simulink model "flightSimulator2"  (R2022a)
settings: Solver=VariableStepAuto  StartTime=0.0  StopTime=10.0  RelTol=1e-3
values from neighbouring files (symbols this model uses):
  g = 9.81    [LQRCalcs.m]    (also in cf_firstOrderStateMdl.m; init_parameters.m; main.m; parameters_buildingSimulink.m)
  Gamma = [cT, cT, cT, cT ... (first row only)    [init_parameters.m]    (also in parameters_buildingSimulink.m; parameters_init.m; parameters_init2.m = [thrustCoeff, thrustCoeff, thrustCoeff, thrustCoeff; parameters_init____CodeToImplementLater.m)
  GammaInv = inv(Gamma)    [init_parameters.m]    (also in parameters_buildingSimulink.m; parameters_init.m)
  J = cat(2, [0 0 0]', J)    [LQRCalcs.m]    (also in init_parameters.m = diag([0.082, 0.0845, 0.1377]); main.m = diag([0.082, 0.0845, 0.1377]); parameters_buildingSimulink.m = diag([0.082, 0.0845, 0.1377]); parameters_init.m = diag([0.082, 0.0845, 0.1377]))
  k_motors = 1    [parameters_buildingSimulink.m]
  k_R = 8.81    [init_parameters.m]    (also in parameters_init____CodeToImplementLater.m)
  Kd_eta = 0    [init_parameters.m]    (also in parameters_buildingSimulink.m)
  Kd_z_eta = 0    [parameters_buildingSimulink.m]
  Kp_eta = 0    [init_parameters.m]    (also in parameters_buildingSimulink.m = 0.5)
  Kp_z_eta = 0.5    [parameters_buildingSimulink.m]
  m = 0.003    [LQRCalcs.m]    (also in cf_firstOrderStateMdl.m; init_parameters.m = 4.34; main.m = 4.34; parameters_buildingSimulink.m = 4.34)
  thrustCoeff = 3.599e-5    (= 3.599e-05)    [parameters_init2.m]
undefined symbols (not defined in the file or in its folder): Gain, k_Omega
libraries: aerolibutil x2, slpidlib x1, matrix_library x1, sharedtransform x1
settings Model: Creator=Drew Lab Computer 1  LastModifiedBy=Drew Lab Computer 1

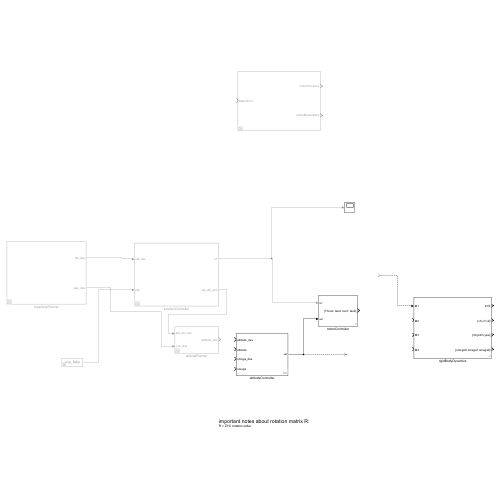
[thumbnail: Simulink's stored preview of the top-level diagram]
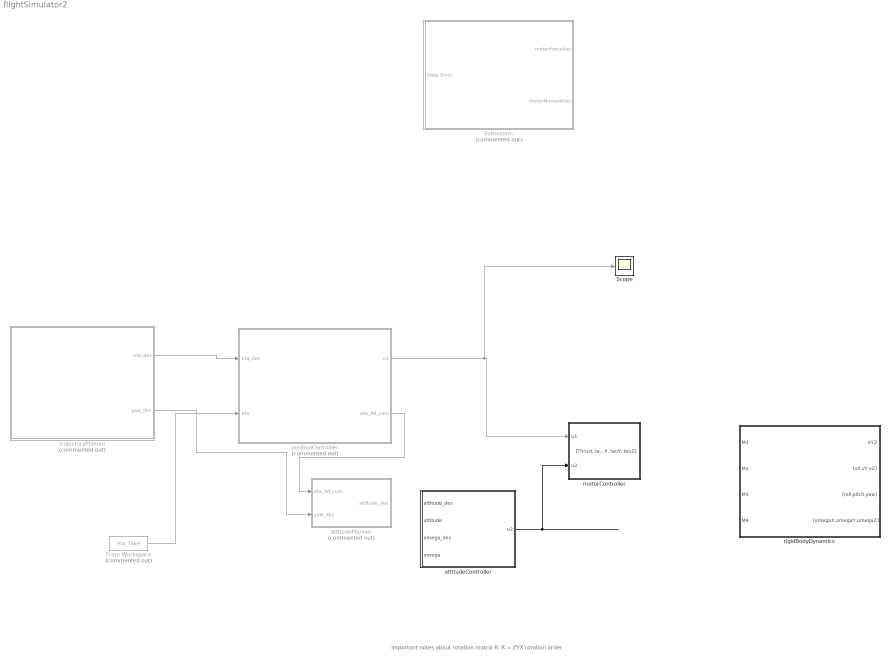
== system flightSimulator2 ==
  note: important notes about rotation matrix R:
      | R = ZYX rotation order
  From Workspace : FromWorkspace  Commented=on  VariableName=eta_fake
  Scope : Scope
  Subsystem : Subsystem  Commented=on
  attitudeController : Subsystem
  attitudePlanner : Subsystem  Commented=on
  motorController : Subsystem
  positionController : Subsystem  Commented=on
  rigidBodyDynamics : Subsystem
  trajectoryPlanner : Subsystem  Commented=on
  wires:
  attitudeController/1(u2) -> motorController/2(u2)
  positionController/1(u1) -> Scope/1, motorController/1(u1)
  trajectoryPlanner/1(eta_des) -> positionController/1(eta_des)
  trajectoryPlanner/2(yaw_des) -> attitudePlanner/2(yaw_des)
  positionController/2(eta_dd_com) -> attitudePlanner/1(eta_dd_com)
  From Workspace/1 -> positionController/2(eta)
  ? -> rigidBodyDynamics/1(M1)

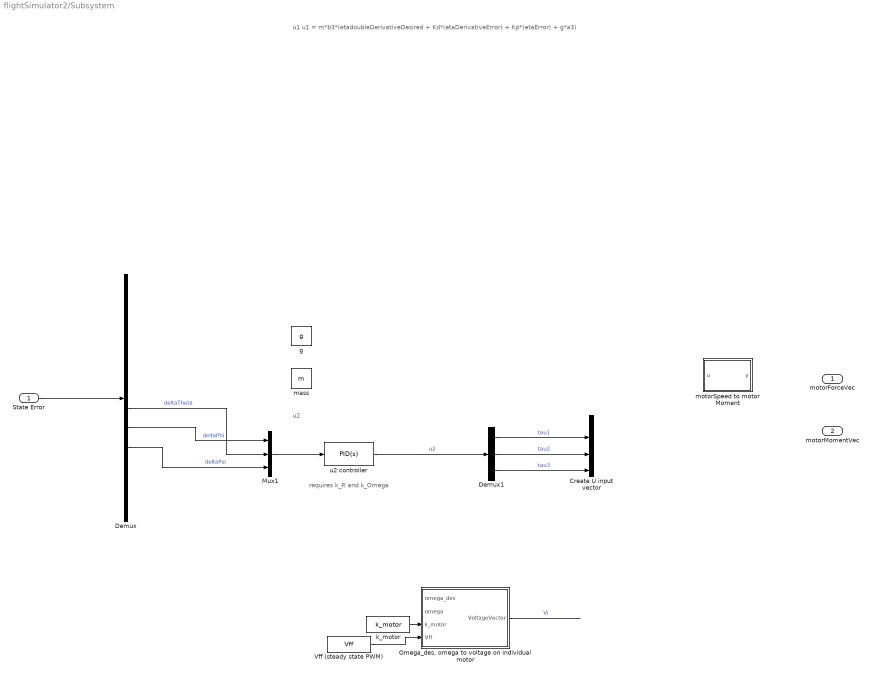
== system flightSimulator2/Subsystem ==
  note: requires k_R and k_Omega
  note: u2
  note: u1
      | u1 = m*b3*(etadoubleDerivativeDesired + Kd*(etaDerivativeError) + Kp*(etaError) + g*a3)
  State Error : Inport
  Create U input vector : Mux
  Demux : Demux  Outputs=12
  Demux1 : Demux  Outputs=3
  Mux1 : Mux  Inputs=3
  "Omega_des, omega to voltage on individual motor" : MATLAB Function  TreatAsAtomicUnit=on
  Vff (steady state PWM) : FromWorkspace  VariableName=Vff
  g : Constant  Value=g
  k_motor : FromWorkspace  VariableName=k_motor
  mass : Constant  Value=m
  motorSpeed to motor Moment : MATLAB Function  TreatAsAtomicUnit=on
  u2 controller : slpidlib/PID Controller  Controller=PID  Form=Parallel  TimeDomain=Continuous-time  UseExternalTs=off  SampleTime=-1  IntegratorMethod=Forward Euler  FilterMethod=Forward Euler  ControllerParametersSource=internal  P=k_R  I=1  UseKiTs=off  D=k_Omega  N=100  UseFilter=on  TunerSelectOption=Transfer Function Based (PID Tuner App)  InitialConditionSource=internal  InitialConditionForIntegrator=0  InitialConditionForFilter=0  DifferentiatorICPrevScaledInput=0  ExternalReset=none  TrackingMode=off  Kt=1  LimitOutput=off  SatLimitsSource=internal  UpperSaturationLimit=inf  LowerSaturationLimit=-inf  LinearizeAsGain=on  AntiWindupMode=none  Kb=1  POutMin=[]  POutMax=[]  IOutMin=[]  IOutMax=[]  DOutMin=[]  DOutMax=[]  NOutMin=[]  NOutMax=[]  SumOutMin=[]  SumOutMax=[]  SaturationOutMin=[]  SaturationOutMax=[]  PParamMin=[]  PParamMax=[]  IParamMin=[]  IParamMax=[]  DParamMin=[]  DParamMax=[]  NParamMin=[]  NParamMax=[]  KbParamMin=[]  KbParamMax=[]  KtParamMin=[]  KtParamMax=[]  KbOutMin=[]  KbOutMax=[]  KtOutMin=[]  KtOutMax=[]  IntegratorOutMin=[]  IntegratorOutMax=[]  FilterOutMin=[]  FilterOutMax=[]  SumI1OutMin=[]  SumI1OutMax=[]  SumI2OutMin=[]  SumI2OutMax=[]  SumI3OutMin=[]  SumI3OutMax=[]  SumI4OutMin=[]  SumI4OutMax=[]  SumDOutMin=[]  SumDOutMax=[]  DifferentiatorOutMin=[]  DifferentiatorOutMax=[]  FilterDiffOutCoefMin=[]  FilterDiffOutCoefMax=[]  ReciprocalOutMin=[]  ReciprocalOutMax=[]  SumDenOutMin=[]  SumDenOutMax=[]  SumNumOutMin=[]  SumNumOutMax=[]  DivideOutMin=[]  DivideOutMax=[]  UdiffTsProdOutMin=[]  UdiffTsProdOutMax=[]  NTsProdOutMin=[]  NTsProdOutMax=[]  UintegralTsProdOutMin=[]  UintegralTsProdOutMax=[]  UngainTsProdOutMin=[]  UngainTsProdOutMax=[]  IntegratorContinuousStateAttributes=''  IntegratorStateMustResolveToSignalObject=off  IntegratorRTWStateStorageClass=Auto  FilterContinuousStateAttributes=''  FilterStateMustResolveToSignalObject=off  FilterRTWStateStorageClass=Auto  ParallelPVariant=InternalParameters  IdealPVariant=Disabled  IVariant=InternalParameters  DVariant=InternalParameters  IntegratorVariant=Continuous  SatVariant=Disabled  AWVariant=Passthrough  PCopyVariant=Disabled  TRVariant=Disabled  FdbkBlocksVariant=Forward  IdealPFdbkVariant=Disabled  SatFdbkVariant=Disabled  DerivativeFilterVariant=ContFilter  NVariant=InternalParameters  NCopyVariant=Disabled  FilterICVariant=InternalICsFilter  IntegratorICVariant=InternalICs  ExternalResetVariant=Disabled  TRSumVariant=Passthrough  SumFdbkVariant=Disabled  SumVariant=Sum_PID  TsampFilterVariant=InternalTs  TsampNgainVariant=Passthrough  TsampIntegralVariant=Passthrough  ExternalSaturationOutDataTypeStr=Inherit: Same as second input  aMode=0
  motorForceVec : Outport
  motorMomentVec : Outport  Port=2
  wires:
  "Omega_des, omega to voltage on individual motor"/1(VoltageVector) -> ?  "Vi"
  State Error/1 -> Demux/1
  Demux/8 -> Mux1/1  "deltaPhi"
  Demux/9 -> Mux1/3  "deltaPsi"
  k_motor/1 -> "Omega_des, omega to voltage on individual motor"/3(k_motor)
  Vff (steady state PWM)/1 -> "Omega_des, omega to voltage on individual motor"/4(Vff)
  Demux/7 -> Mux1/2  "deltaTheta"
  Mux1/1 -> u2 controller/1
  u2 controller/1 -> Demux1/1  "u2"
  ? -> Create U input vector/1  "thrustSum"
  Demux1/3 -> Create U input vector/4  "tau3"
  Demux1/2 -> Create U input vector/3  "tau2"
  Demux1/1 -> Create U input vector/2  "tau1"

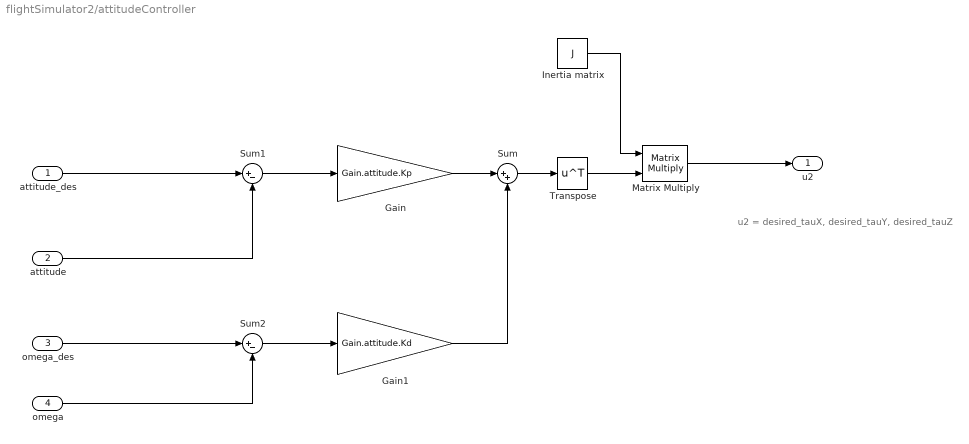
== system flightSimulator2/attitudeController ==
  note: u2 = desired_tauX, desired_tauY, desired_tauZ
  attitude_des : Inport
  attitude : Inport  Port=2
  omega_des : Inport  Port=3
  omega : Inport  Port=4
  Gain : Gain  Gain=Gain.attitude.Kp
  Gain1 : Gain  Gain=Gain.attitude.Kd
  Inertia matrix : Constant  Value=J
  Matrix Multiply : Product  Multiplication=Matrix(*)
  Sum : Sum  Inputs=|++
  Sum1 : Sum  Inputs=|+-
  Sum2 : Sum  Inputs=|+-
  Transpose : Math  Operator=transpose
  u2 : Outport
  wires:
  attitude_des/1 -> Sum1/1
  attitude/1 -> Sum1/2
  omega_des/1 -> Sum2/1
  omega/1 -> Sum2/2
  Sum1/1 -> Gain/1
  Gain/1 -> Sum/1
  Sum2/1 -> Gain1/1
  Gain1/1 -> Sum/2
  Inertia matrix/1 -> Matrix Multiply/1
  Sum/1 -> Transpose/1
  Transpose/1 -> Matrix Multiply/2
  Matrix Multiply/1 -> u2/1

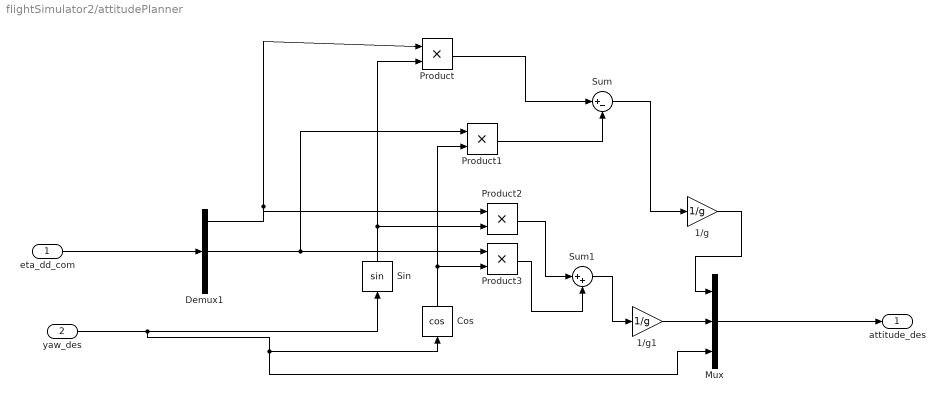
== system flightSimulator2/attitudePlanner ==
  eta_dd_com : Inport
  yaw_des : Inport  Port=2
  1/g : Gain  Gain=1/g
  1/g1 : Gain  Gain=1/g
  Cos : Trigonometry  Operator=cos
  Demux1 : Demux  Outputs=3
  Mux : Mux  Inputs=3
  Product{,1..3} (4 alike) : Product
  Sin : Trigonometry
  Sum : Sum  Inputs=|+-
  Sum1 : Sum  Inputs=|++
  attitude_des : Outport
  wires:
  Mux/1 -> attitude_des/1
  eta_dd_com/1 -> Demux1/1
  yaw_des/1 -> Sin/1, Cos/1, Mux/3
  Sum1/1 -> 1/g1/1
  1/g/1 -> Mux/1
  Demux1/1 -> Product/1, Product2/1
  Sin/1 -> Product/2, Product2/2
  Cos/1 -> Product1/2, Product3/2
  Demux1/2 -> Product1/1, Product3/1
  Product/1 -> Sum/1
  Product1/1 -> Sum/2
  Sum/1 -> 1/g/1
  1/g1/1 -> Mux/2
  Product2/1 -> Sum1/1
  Product3/1 -> Sum1/2

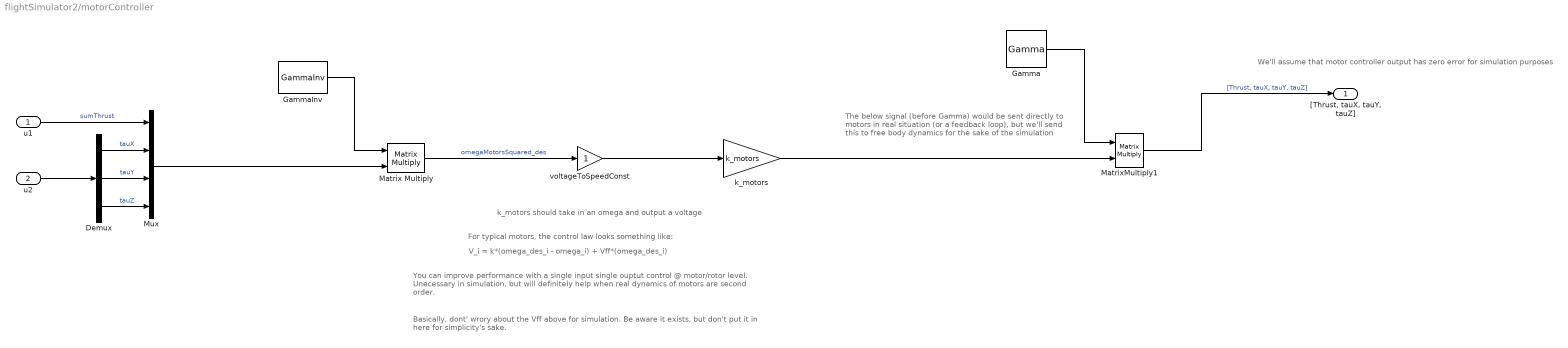
== system flightSimulator2/motorController ==
  note: We'll assume that motor controller output has zero error for simulation purposes
  note: The below signal (before Gamma) would be sent directly to motors in real situation (or a feedback loop), but we'll send this to free body dynamics for the sake of the simulation
  note: k_motors should take in an omega and output a voltage
  note: Basically, dont' wrory about the Vff above for simulation. Be aware it exists, but don't put it in here for simplicity's sake.
  note: You can improve performance with a single input single ouptut control @ motor/rotor level. Unecessary in simulation, but will definitely help when real dynamics of motors are second order.
  note: V_i = k*(omega_des_i - omega_i) + Vff*(omega_des_i)
  note: For typical motors, the control law looks something like:
  u1 : Inport
  u2 : Inport  Port=2
  Demux : Demux  Outputs=3
  Gamma : Constant  Value=Gamma
  GammaInv : Constant  Value=GammaInv
  Matrix Multiply : Product  Multiplication=Matrix(*)
  MatrixMultiply1 : Product  Multiplication=Matrix(*)
  Mux : Mux
  k_motors : Gain  Gain=k_motors
  voltageToSpeedConst : Gain
  "[Thrust, tauX, tauY, tauZ]" : Outport
  wires:
  u2/1 -> Demux/1
  u1/1 -> Mux/1  "sumThrust"
  Demux/2 -> Mux/3  "tauY"
  Demux/1 -> Mux/2  "tauX"
  Demux/3 -> Mux/4  "tauZ"
  Gamma/1 -> MatrixMultiply1/1
  MatrixMultiply1/1 -> "[Thrust, tauX, tauY, tauZ]"/1  "[Thrust, tauX, tauY, tauZ]"
  Mux/1 -> Matrix Multiply/2
  GammaInv/1 -> Matrix Multiply/1
  Matrix Multiply/1 -> voltageToSpeedConst/1  "omegaMotorsSquared_des"
  voltageToSpeedConst/1 -> k_motors/1
  k_motors/1 -> MatrixMultiply1/2

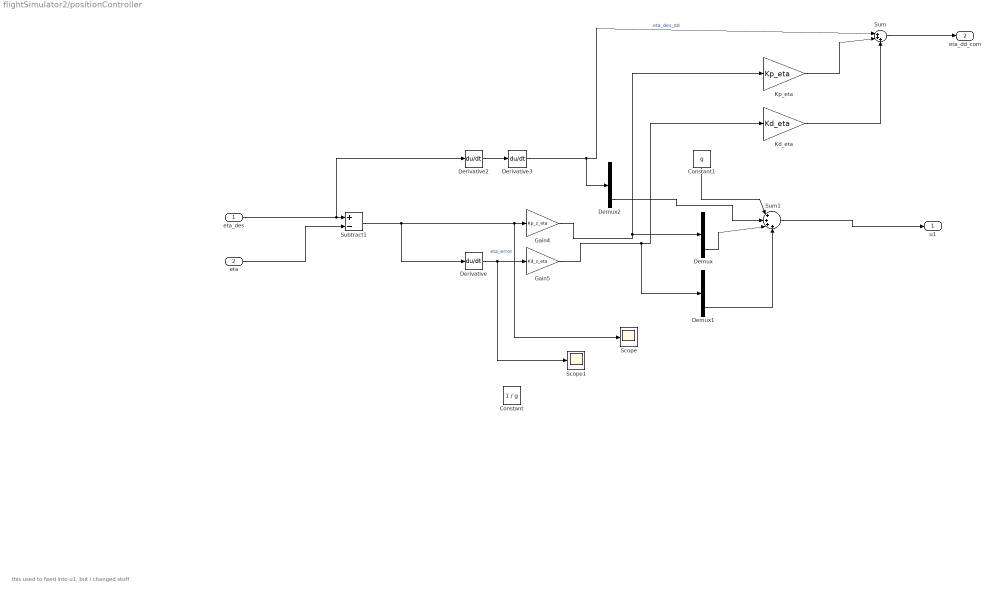
== system flightSimulator2/positionController ==
  note: this used to feed into u1, but i changed stuff
  eta_des : Inport
  eta : Inport  Port=2
  Constant : Constant  Value=1 / g
  Constant1 : Constant  Value=g
  Demux : Demux  Outputs=3
  Demux1 : Demux  Outputs=3
  Demux2 : Demux  Outputs=3
  Derivative : Derivative
  Derivative2 : Derivative
  Derivative3 : Derivative
  Gain4 : Gain  Gain=Kp_z_eta
  Gain5 : Gain  Gain=Kd_z_eta
  Kd_eta : Gain  Gain=Kd_eta
  Kp_eta : Gain  Gain=Kp_eta
  Scope : Scope
  Scope1 : Scope
  Subtract1 : Sum  Inputs=+-
  Sum : Sum  Inputs=|+++
  Sum1 : Sum  Inputs=|++++
  u1 : Outport
  eta_dd_com : Outport  Port=2
  wires:
  eta_des/1 -> Derivative2/1, Subtract1/1
  eta/1 -> Subtract1/2
  Subtract1/1 -> Derivative/1, Scope/1, Gain4/1  "eta_error"
  Derivative/1 -> Scope1/1, Gain5/1
  Gain4/1 -> Kp_eta/1, Demux/1
  Gain5/1 -> Demux1/1, Kd_eta/1
  Sum1/1 -> u1/1
  Derivative2/1 -> Derivative3/1
  Derivative3/1 -> Demux2/1, Sum/1  "eta_des_dd"
  Constant1/1 -> Sum1/1
  Kp_eta/1 -> Sum/2
  Kd_eta/1 -> Sum/3
  Sum/1 -> eta_dd_com/1
  Demux2/3 -> Sum1/2
  Demux/3 -> Sum1/3
  Demux1/3 -> Sum1/4

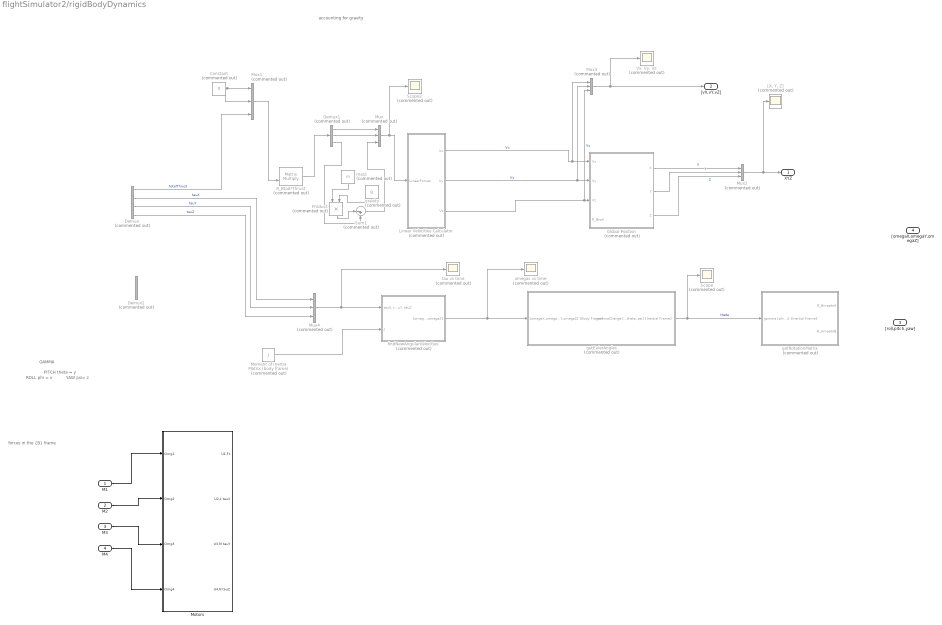
== system flightSimulator2/rigidBodyDynamics ==
  note: GAMMA
  note: accounting for gravity
  note: forces in the {B} frame
  note: ROLL
      | phi = x
  note: PITCH
      | theta = y
  note: YAW
      | psi= z
  M1 : Inport
  M2 : Inport  Port=2
  M3 : Inport  Port=3
  M4 : Inport  Port=4
  Constant : Constant  Commented=on  Value=0
  Demux : Demux  Commented=on
  Demux1 : Demux  Commented=on  Outputs=3
  Demux2 : Demux  Commented=on  Outputs=3
  Global Position : Subsystem  Commented=on
  Linear Velocities Calculator : Subsystem  Commented=on
  Moment of Inertia Matrix (body frame) : Constant  Commented=on  Value=J  VectorParams1D=off
  Motors : Subsystem
  Mux{,1..4} (5 alike) : Mux  Commented=on  Inputs=3
  Product : Product  Commented=on
  R_BtoA*Thrust : Product  Commented=on  Multiplication=Matrix(*)
  Scope : Scope  Commented=on
  Scope2 : Scope  Commented=on
  Sum1 : Sum  Commented=on  Inputs=|-+
  "Vx, Vy, Vz" : Scope  Commented=on
  "[X, Y, Z]" : Scope  Commented=on
  findNewAngularVelocities : Subsystem  Commented=on
  getEulerAngles : Subsystem  Commented=on
  getRotationMatrix : Subsystem  Commented=on
  gravity : Constant  Commented=on  Value=g
  mass : Constant  Commented=on  Value=m
  omegas vs time : Scope  Commented=on
  tau vs time : Scope  Commented=on
  XYZ : Outport
  "[vX,vY,vZ]" : Outport  Port=2
  "[roll,pitch,yaw]" : Outport  Port=3
  "[omegaX,omegaY,omegaZ]" : Outport  Port=4
  wires:
  mass/1 -> Product/1
  Product/1 -> Sum1/1
  Mux/1 -> Scope2/1, Linear Velocities Calculator/1(LinearForces)
  Linear Velocities Calculator/3(Vz) -> Mux3/3, Global Position/3(Vz)  "Vz"
  Mux1/1 -> R_BtoA*Thrust/2
  Linear Velocities Calculator/1(Vx) -> Mux3/1, Global Position/1(Vx)  "Vx"
  R_BtoA*Thrust/1 -> Demux1/1
  Demux/2 -> Mux4/1  "tauX"
  Demux/4 -> Mux4/3  "tauZ"
  Demux/3 -> Mux4/2  "tauY"
  Constant/1 -> Mux1/2, Mux1/1
  Linear Velocities Calculator/2(Vy) -> Mux3/2, Global Position/2(Vy)  "Vy"
  Demux1/2 -> Mux/2
  gravity/1 -> Product/2
  Sum1/1 -> Mux/3
  Demux/1 -> Mux1/3  "totalThrust"
  Demux1/3 -> Sum1/2
  Demux1/1 -> Mux/1
  Global Position/2(Y) -> Mux2/2  "Y"
  Global Position/3(Z) -> Mux2/3  "Z"
  Global Position/1(X) -> Mux2/1  "X"
  Mux2/1 -> "[X, Y, Z]"/1, XYZ/1
  Mux3/1 -> "Vx, Vy, Vz"/1, "[vX,vY,vZ]"/1
  Mux4/1 -> tau vs time/1, findNewAngularVelocities/1("tauX, tauY, tauZ")
  Moment of Inertia Matrix (body frame)/1 -> findNewAngularVelocities/2(J)
  findNewAngularVelocities/1("[omegaX,omegaY,omegaZ]") -> omegas vs time/1, getEulerAngles/1("[omegaX,omegaY,omegaZ] {Body Frame}")
  getEulerAngles/1("gammaChange [phi, theta, psi] {Inertial Frame}") -> getRotationMatrix/1("gamma [phi, theta, psi] {Inertial Frame}"), Scope/1  "theta"
  M2/1 -> Motors/2(Omg2)
  M3/1 -> Motors/3(Omg3)
  M1/1 -> Motors/1(Omg1)
  M4/1 -> Motors/4(Omg4)

== system flightSimulator2/trajectoryPlanner ==
  From Workspace : FromWorkspace  VariableName=eta_des
  From Workspace1 : FromWorkspace  VariableName=yaw_des
  eta_des : Outport
  yaw_des : Outport  Port=2
  wires:
  From Workspace/1 -> eta_des/1
  From Workspace1/1 -> yaw_des/1

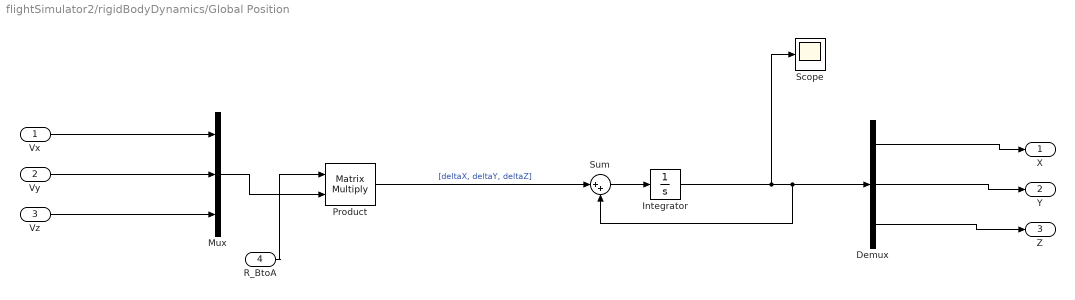
== system flightSimulator2/rigidBodyDynamics/Global Position ==
  Vx : Inport
  Vy : Inport  Port=2
  Vz : Inport  Port=3
  R_BtoA : Inport  Port=4
  Demux : Demux  Outputs=3
  Integrator : Integrator
  Mux : Mux  Inputs=3
  Product : Product  Multiplication=Matrix(*)
  Scope : Scope
  Sum : Sum  Inputs=|++
  X : Outport
  Y : Outport  Port=2
  Z : Outport  Port=3
  wires:
  Demux/2 -> Y/1
  Demux/1 -> X/1
  Demux/3 -> Z/1
  Vz/1 -> Mux/3
  Vy/1 -> Mux/2
  Vx/1 -> Mux/1
  R_BtoA/1 -> Product/1
  Product/1 -> Sum/1  "[deltaX, deltaY, deltaZ]"
  Integrator/1 -> Demux/1, Sum/2, Scope/1
  Sum/1 -> Integrator/1
  Mux/1 -> Product/2

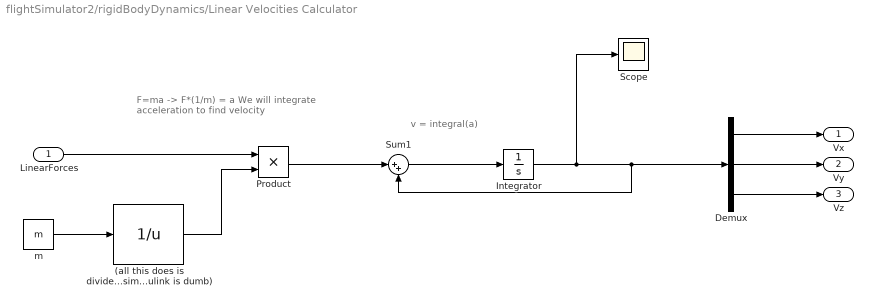
== system flightSimulator2/rigidBodyDynamics/Linear Velocities Calculator ==
  note: v = integral(a)
  note: F=ma -> F*(1/m) = a
      | We will integrate acceleration to find velocity
  LinearForces : Inport
  (all this does is divide...simulink is dumb) : Math  Operator=reciprocal  SignedPower=on
  Demux : Demux  Outputs=3
  Integrator : Integrator
  Product : Product
  Scope : Scope
  Sum1 : Sum  Inputs=|++
  m : Constant  Value=m
  Vx : Outport
  Vy : Outport  Port=2
  Vz : Outport  Port=3
  wires:
  LinearForces/1 -> Product/1
  m/1 -> (all this does is divide...simulink is dumb)/1
  (all this does is divide...simulink is dumb)/1 -> Product/2
  Demux/1 -> Vx/1
  Demux/2 -> Vy/1
  Demux/3 -> Vz/1
  Integrator/1 -> Scope/1, Demux/1, Sum1/2
  Product/1 -> Sum1/1
  Sum1/1 -> Integrator/1

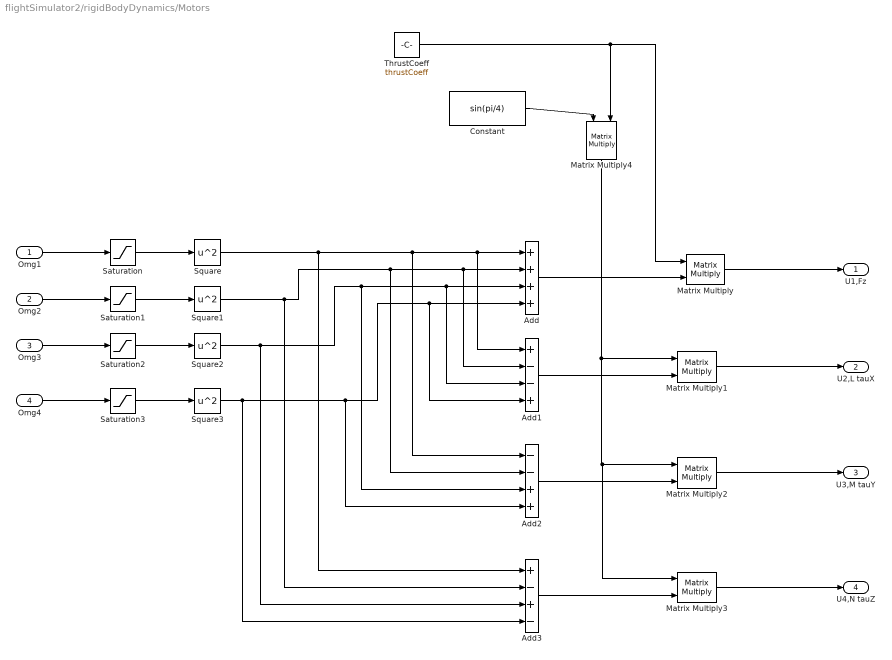
== system flightSimulator2/rigidBodyDynamics/Motors ==
  Omg1 : Inport
  Omg2 : Inport  Port=2
  Omg3 : Inport  Port=3
  Omg4 : Inport  Port=4
  Add : Sum  Inputs=++++
  Add1 : Sum  Inputs=+--+
  Add2 : Sum  Inputs=--++
  Add3 : Sum  Inputs=+-+-
  Constant : Constant  Value=sin(pi/4)
  Matrix Multiply{,1..4} (5 alike) : Product  Multiplication=Matrix(*)
  Saturation{,1..3} (4 alike) : Saturate
  Square{,1..3} (4 alike) : Math  Operator=square
  ThrustCoeff : Constant  Value=thrustCoeff
  U1,Fz : Outport
  U2,L tauX : Outport  Port=2
  U3,M tauY : Outport  Port=3
  U4,N tauZ : Outport  Port=4
  wires:
  Omg1/1 -> Saturation/1
  Omg2/1 -> Saturation1/1
  Omg3/1 -> Saturation2/1
  Omg4/1 -> Saturation3/1
  Saturation/1 -> Square/1
  Saturation1/1 -> Square1/1
  Saturation2/1 -> Square2/1
  Saturation3/1 -> Square3/1
  Square/1 -> Add3/1, Add2/1, Add1/1, Add/1
  Square1/1 -> Add3/2, Add2/2, Add1/2, Add/2
  Square2/1 -> Add3/3, Add2/3, Add1/3, Add/3
  Square3/1 -> Add3/4, Add2/4, Add1/4, Add/4
  Add/1 -> Matrix Multiply/2
  ThrustCoeff/1 -> Matrix Multiply/1, Matrix Multiply4/2
  Add1/1 -> Matrix Multiply1/2
  Add2/1 -> Matrix Multiply2/2
  Add3/1 -> Matrix Multiply3/2
  Constant/1 -> Matrix Multiply4/1
  Matrix Multiply4/1 -> Matrix Multiply3/1, Matrix Multiply2/1, Matrix Multiply1/1
  Matrix Multiply/1 -> U1,Fz/1
  Matrix Multiply1/1 -> U2,L tauX/1
  Matrix Multiply2/1 -> U3,M tauY/1
  Matrix Multiply3/1 -> U4,N tauZ/1

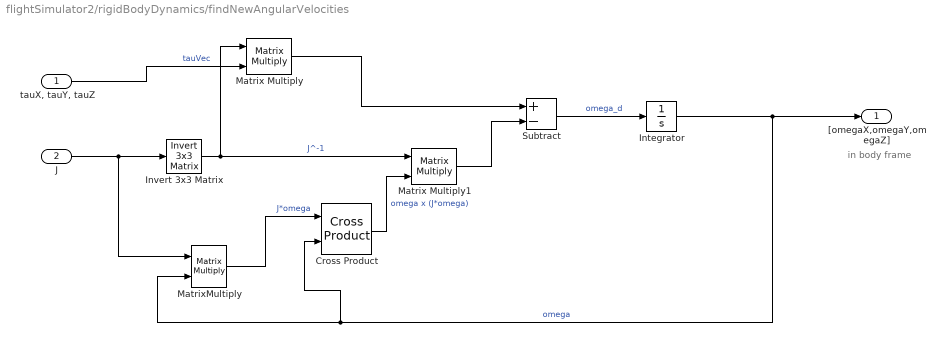
== system flightSimulator2/rigidBodyDynamics/findNewAngularVelocities ==
  note: in body frame
  "tauX, tauY, tauZ" : Inport
  J : Inport  Port=2
  Cross Product : matrix_library/Cross Product
      settings: SourceProductBaseCode=SL
  Integrator : Integrator
  Invert 3x3 Matrix : aerolibutil/Invert  3x3 Matrix
  Matrix Multiply : Product  Multiplication=Matrix(*)
  Matrix Multiply1 : Product  Multiplication=Matrix(*)
  MatrixMultiply : Product  Multiplication=Matrix(*)
  Subtract : Sum  Inputs=+-
  "[omegaX,omegaY,omegaZ]" : Outport
  wires:
  J/1 -> MatrixMultiply/1, Invert 3x3 Matrix/1
  Subtract/1 -> Integrator/1  "omega_d"
  Integrator/1 -> Cross Product/2, MatrixMultiply/2, "[omegaX,omegaY,omegaZ]"/1  "omega"
  Invert 3x3 Matrix/1 -> Matrix Multiply1/1, Matrix Multiply/1  "J^-1"
  "tauX, tauY, tauZ"/1 -> Matrix Multiply/2  "tauVec"
  Matrix Multiply/1 -> Subtract/1
  MatrixMultiply/1 -> Cross Product/1  "J*omega"
  Cross Product/1 -> Matrix Multiply1/2  "omega x (J*omega)"
  Matrix Multiply1/1 -> Subtract/2

== system flightSimulator2/rigidBodyDynamics/getEulerAngles ==
  "[omegaX,omegaY,omegaZ] {Body Frame}" : Inport
  Integrator : Integrator
  "gammaChange [phi, theta, psi] {Inertial Frame}" : Outport
  wires:
  "[omegaX,omegaY,omegaZ] {Body Frame}"/1 -> Integrator/1
  Integrator/1 -> "gammaChange [phi, theta, psi] {Inertial Frame}"/1

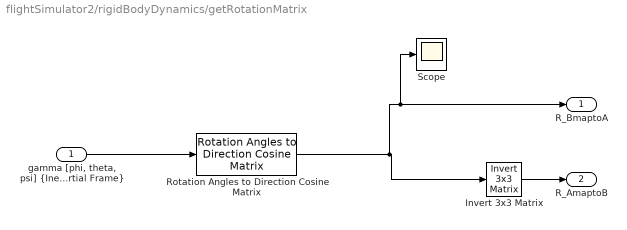
== system flightSimulator2/rigidBodyDynamics/getRotationMatrix ==
  "gamma [phi, theta, psi] {Inertial Frame}" : Inport
  Invert 3x3 Matrix : aerolibutil/Invert  3x3 Matrix
  Rotation Angles to Direction Cosine Matrix : sharedtransform/Rotation Angles to Direction Cosine Matrix  rotationOrder=ZYX  aMode=aMode
      settings: SourceProductBaseCode=AE,PW,DR,MT,VE
  Scope : Scope
  R_BmaptoA : Outport
  R_AmaptoB : Outport  Port=2
  wires:
  "gamma [phi, theta, psi] {Inertial Frame}"/1 -> Rotation Angles to Direction Cosine Matrix/1
  Rotation Angles to Direction Cosine Matrix/1 -> Scope/1, R_BmaptoA/1, Invert 3x3 Matrix/1
  Invert 3x3 Matrix/1 -> R_AmaptoB/1

== matlab function flightSimulator2/Subsystem/motorSpeed to motor Moment ==
  data: u input; y output
function y = fcn(u)

y = u;

== matlab function flightSimulator2/Subsystem/Omega_des, omega to voltage on individual motor ==
  data: omega_des input; VoltageVector output; omega input; k_motor input; Vff input
function VoltageVector = fcn(omega_des, omega, k_motor, Vff)
% omega_des = [omega1, omega2, omega3, omega4]
% omega = [omega1, omega2, omega3, omega4]
[r, c] = size(omega)
omegaLen = max([r, c]) % picks whatever direction omega is in 
for i=[1:omegaLen]
    VoltageVector(i) = k_motor.*(omega_des(i) - omega(i)) + Vff.*(omega_des(i));

    
end
VoltageVector = VoltageVector'; %Formats V as a column vector output
